simulink model "example1_simul"  (R2018a)
settings: Solver=VariableStepAuto  StartTime=0.0  StopTime=0.02  RelTol=1e-3
values from neighbouring files (symbols this model uses):
  Am = [-R1/L1 0 -1/L1;      0 -R2/L2 1/L2;      1/C -1/C 0]    [example1_params.m]
  Bm = [1/L1; 0; 0]    [example1_params.m]
  C = 250e-6    (= 0.00025)    [example1_params.m]
  Cm = [0 R2 0]    [example1_params.m]
  Dm = 0    [example1_params.m]
  L1 = 1e-3    (= 0.001)    [example1_params.m]
  L2 = 2e-3    (= 0.002)    [example1_params.m]
  R1 = 1    [example1_params.m]
  R2 = 100    [example1_params.m]
settings Model: Creator=gbecerra  LastModifiedBy=gbecerra

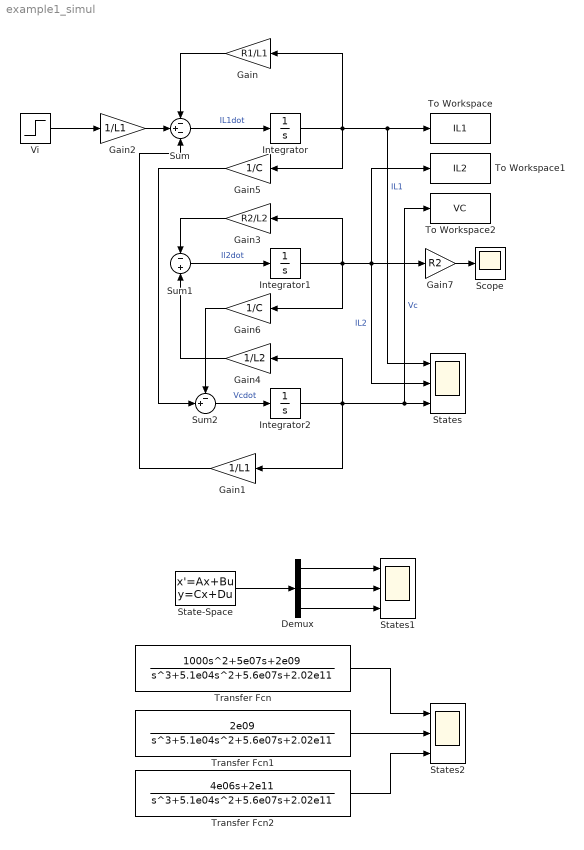
== system example1_simul ==
  Demux : Demux  Outputs=3
  Gain : Gain  Gain=R1/L1
  Gain1 : Gain  Gain=1/L1
  Gain2 : Gain  Gain=1/L1
  Gain3 : Gain  Gain=R2/L2
  Gain4 : Gain  Gain=1/L2
  Gain5 : Gain  Gain=1/C
  Gain6 : Gain  Gain=1/C
  Gain7 : Gain  Gain=R2
  Integrator : Integrator
  Integrator1 : Integrator
  Integrator2 : Integrator
  Scope : Scope
  State-Space : StateSpace  A=Am  B=Bm  C=Cm  D=Dm  InitialCondition=0
  States : Scope  NumInputPorts=3
  States1 : Scope  NumInputPorts=3
  States2 : Scope  NumInputPorts=3
  Sum : Sum  Inputs=-+-
  Sum1 : Sum  Inputs=-|+
  Sum2 : Sum  Inputs=-+|
  To Workspace : ToWorkspace  VariableName=IL1  SaveFormat=Timeseries  SampleTime=-1
  To Workspace1 : ToWorkspace  VariableName=IL2  SaveFormat=Timeseries  SampleTime=-1
  To Workspace2 : ToWorkspace  VariableName=VC  SaveFormat=Timeseries  SampleTime=-1
  Transfer Fcn : TransferFcn  Numerator=[1000 5e07 2e09]  Denominator=[1 5.1e04 5.6e07 2.02e11]
  Transfer Fcn1 : TransferFcn  Numerator=2e09  Denominator=[1 5.1e04 5.6e07 2.02e11]
  Transfer Fcn2 : TransferFcn  Numerator=[4e06 2e11]  Denominator=[1 5.1e04 5.6e07 2.02e11]
  Vi : Step  Time=0.002  SampleTime=0
  wires:
  Integrator/1 -> Gain5/1, To Workspace/1, States/1, Gain/1  "IL1"
  Sum/1 -> Integrator/1  "IL1dot"
  Integrator1/1 -> Gain7/1, To Workspace1/1, States/2, Gain3/1, Gain6/1  "IL2"
  Integrator2/1 -> Gain4/1, To Workspace2/1, States/3, Gain1/1  "Vc"
  Sum1/1 -> Integrator1/1  "Il2dot"
  Sum2/1 -> Integrator2/1  "Vcdot"
  Gain/1 -> Sum/1
  Gain1/1 -> Sum/3
  Gain2/1 -> Sum/2
  Gain3/1 -> Sum1/1
  Gain4/1 -> Sum1/2
  Gain5/1 -> Sum2/2
  Gain6/1 -> Sum2/1
  Gain7/1 -> Scope/1
  Vi/1 -> Gain2/1
  State-Space/1 -> Demux/1
  Demux/1 -> States1/1
  Demux/2 -> States1/2
  Demux/3 -> States1/3
  Transfer Fcn1/1 -> States2/2
  Transfer Fcn/1 -> States2/1
  Transfer Fcn2/1 -> States2/3
